simulink model "Global_Nocontrol"  (R2016a)
settings: Solver=ode8  StartTime=0.0  StopTime=1400  FixedStep=1  RelTol=1e-3
(part 1 of 2)
settings Model: Creator=Abhiram  LastModifiedBy=Abhiram
settings GRTTargetCC: GeneratePreprocessorConditionals=Use local settings

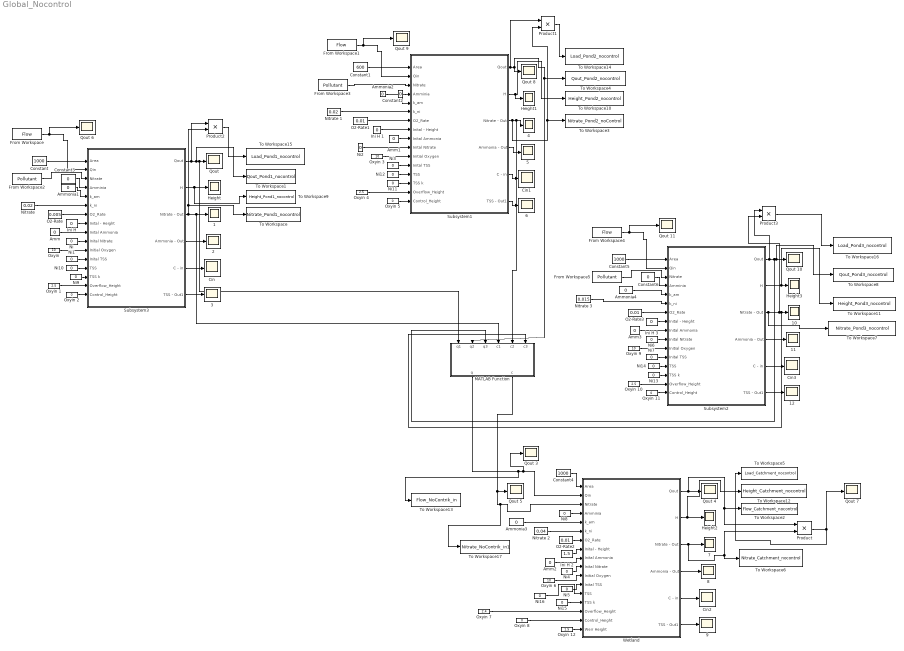
== system Global_Nocontrol ==
   Amm{,1..3} (4 alike) : Constant  Value=0
  {1..12} (12 alike) : Scope
  Ammonia{1..4} (4 alike) : Constant  Value=0
  Cin{,1..3} (4 alike) : Scope
  Constant : Constant  Value=1000
  Constant1 : Constant  Value=600
  Constant2 : Constant  Value=0
  Constant3 : Constant  Value=0
  Constant4 : Constant  Value=1000
  Constant5 : Constant  Value=1000
  Constant6 : Constant  Value=0
  From Workspace : FromWorkspace  VariableName=Flow  SampleTime=0
  From Workspace1 : FromWorkspace  VariableName=Flow  SampleTime=0
  From Workspace2 : FromWorkspace  VariableName=Pollutant  SampleTime=0
  From Workspace3 : FromWorkspace  VariableName=Pollutant  SampleTime=0
  From Workspace4 : FromWorkspace  VariableName=Flow  SampleTime=0
  From Workspace5 : FromWorkspace  VariableName=Pollutant  SampleTime=0
  Height{,1..3} (4 alike) : Scope
  "Ini H " : Constant  Value=0
  Ini H 1 : Constant  Value=0
  Ini H 2 : Constant  Value=1.5
  Ini H 3 : Constant  Value=0
  MATLAB Function : MATLAB Function  TreatAsAtomicUnit=on
  Ni{,1..16} (17 alike) : Constant  Value=0
  "Nitrate " : Constant  Value=0.02
  Nitrate 1 : Constant  Value=0.02
  Nitrate 2 : Constant  Value=0.04
  Nitrate 3 : Constant  Value=0.015
  O2-Rate : Constant  Value=0.005
  O2-Rate1 : Constant  Value=0.01
  O2-Rate2 : Constant  Value=0.01
  O2-Rate3 : Constant  Value=0.01
  Oxyin {,3,6,9} (4 alike) : Constant  Value=10
  Oxyin 1 : Constant  Value=2.5
  Oxyin 10 : Constant  Value=2.5
  Oxyin {2,5,8,11} (4 alike) : Constant  Value=0
  Oxyin 12 : Constant  Value=1.5
  Oxyin 4 : Constant  Value=2.5
  Oxyin 7 : Constant  Value=2.4
  Product{,1..3} (4 alike) : Product
  Qout {,3..11} (10 alike) : Scope
  Subsystem1 : Subsystem
  Subsystem2 : Subsystem
  Subsystem3 : Subsystem
  To Workspace : ToWorkspace  VariableName=Nitrate_Pond1_nocontrol  SampleTime=-1
      settings: Save2DSignal=2-D array (concatenate along first dimension)
  To Workspace1 : ToWorkspace  VariableName=Qout_Pond1_nocontrol  SampleTime=-1
      settings: Save2DSignal=2-D array (concatenate along first dimension)
  To Workspace10 : ToWorkspace  VariableName=Height_Pond2_nocontrol  SampleTime=-1
      settings: Save2DSignal=2-D array (concatenate along first dimension)
  To Workspace11 : ToWorkspace  VariableName=Height_Pond3_nocontrol  SampleTime=-1
      settings: Save2DSignal=2-D array (concatenate along first dimension)
  To Workspace12 : ToWorkspace  VariableName=Height_Catchment_nocontrol  SampleTime=-1
      settings: Save2DSignal=2-D array (concatenate along first dimension)
  To Workspace13 : ToWorkspace  VariableName=Flow_NoContrik_in  SampleTime=-1
      settings: Save2DSignal=2-D array (concatenate along first dimension)
  To Workspace14 : ToWorkspace  VariableName=Load_Pond2_nocontrol  SampleTime=-1
      settings: Save2DSignal=2-D array (concatenate along first dimension)
  To Workspace15 : ToWorkspace  VariableName=Load_Pond1_nocontrol  SampleTime=-1
      settings: Save2DSignal=2-D array (concatenate along first dimension)
  To Workspace16 : ToWorkspace  VariableName=Load_Pond3_nocontrol  SampleTime=-1
      settings: Save2DSignal=2-D array (concatenate along first dimension)
  To Workspace17 : ToWorkspace  VariableName=Nitrate_NoContrik_in1  SampleTime=-1
      settings: Save2DSignal=2-D array (concatenate along first dimension)
  To Workspace2 : ToWorkspace  VariableName=Flow_Catchment_nocontrol  SampleTime=-1
      settings: Save2DSignal=2-D array (concatenate along first dimension)
  To Workspace3 : ToWorkspace  VariableName=Nitrate_Pond2_noControl  SampleTime=-1
      settings: Save2DSignal=2-D array (concatenate along first dimension)
  To Workspace4 : ToWorkspace  VariableName=Qout_Pond2_nocontrol  SampleTime=-1
      settings: Save2DSignal=2-D array (concatenate along first dimension)
  To Workspace5 : ToWorkspace  VariableName=Load_Catchment_nocontrol  SampleTime=-1
      settings: Save2DSignal=2-D array (concatenate along first dimension)
  To Workspace6 : ToWorkspace  VariableName=Nitrate_Catchment_nocontrol  SampleTime=-1
      settings: Save2DSignal=2-D array (concatenate along first dimension)
  To Workspace7 : ToWorkspace  VariableName=Nitrate_Pond3_nocontrol  SampleTime=-1
      settings: Save2DSignal=2-D array (concatenate along first dimension)
  To Workspace8 : ToWorkspace  VariableName=Qout_Pond3_nocontrol  SampleTime=-1
      settings: Save2DSignal=2-D array (concatenate along first dimension)
  To Workspace9 : ToWorkspace  VariableName=Height_Pond1_nocontrol  SampleTime=-1
      settings: Save2DSignal=2-D array (concatenate along first dimension)
  Wetland : Subsystem
  wires:
  "Nitrate "/1 -> Subsystem3/6(k_ni)
  Constant/1 -> Subsystem3/1(Area)
  Ammonia1/1 -> Subsystem3/5(k_am)
  From Workspace2/1 -> Subsystem3/3(Nitrate)
  Constant3/1 -> Subsystem3/4(Amminia)
  O2-Rate/1 -> Subsystem3/7("O2_Rate ")
  Subsystem3/5("C - in ") -> Cin/1
  "Ini H "/1 -> Subsystem3/8(Inital - Height)
  " Amm"/1 -> Subsystem3/9(Inital Ammonia)
  Ni/1 -> Subsystem3/10(Inital Nitrate)
  "Oxyin "/1 -> Subsystem3/11(Initial Oxygen)
  Subsystem3/6(TSS - Out1) -> 3/1
  Ni1/1 -> Subsystem3/12(Inital TSS)
  From Workspace/1 -> Subsystem3/2(Qin), Qout 6/1
  Oxyin 1/1 -> Subsystem3/15(Overflow_Height)
  Oxyin 2/1 -> Subsystem3/16(Control_Height)
  Subsystem3/4(Ammonia - Out) -> 2/1
  Nitrate 2/1 -> Wetland/6(k_ni)
  Constant4/1 -> Wetland/1(Area)
  Ammonia3/1 -> Wetland/5(k_am)
  O2-Rate2/1 -> Wetland/7("O2_Rate ")
  Wetland/4(Ammonia - Out) -> 8/1
  Wetland/5("C - in ") -> Cin2/1
  Ini H 2/1 -> Wetland/8(Inital - Height)
  " Amm2"/1 -> Wetland/9(Inital Ammonia)
  Ni4/1 -> Wetland/10(Inital Nitrate)
  Oxyin 6/1 -> Wetland/11(Initial Oxygen)
  Wetland/6(TSS - Out1) -> 9/1
  Ni5/1 -> Wetland/12(Inital TSS)
  Oxyin 7/1 -> Wetland/15(Overflow_Height)
  Oxyin 8/1 -> Wetland/16(Control_Height)
  Wetland/3(Nitrate - Out) -> 7/1, Product/2, To Workspace6/1
  Wetland/1(Qout) -> Product/1, To Workspace2/1, Qout 4/1
  Product/1 -> Qout 7/1, To Workspace5/1
  MATLAB Function/2(c) -> To Workspace17/1, Wetland/3(Nitrate), Qout 5/1
  Ni8/1 -> Wetland/4(Amminia)
  Oxyin 12/1 -> Wetland/17(Weir Height)
  Nitrate 1/1 -> Subsystem1/6(k_ni)
  Constant1/1 -> Subsystem1/1(Area)
  Ammonia2/1 -> Subsystem1/5(k_am)
  From Workspace3/1 -> Subsystem1/3(Nitrate)
  Constant2/1 -> Subsystem1/4(Amminia)
  O2-Rate1/1 -> Subsystem1/7("O2_Rate ")
  Subsystem1/5("C - in ") -> Cin1/1
  Ini H 1/1 -> Subsystem1/8(Inital - Height)
  " Amm1"/1 -> Subsystem1/9(Inital Ammonia)
  Ni2/1 -> Subsystem1/10(Inital Nitrate)
  Oxyin 3/1 -> Subsystem1/11(Initial Oxygen)
  Subsystem1/6(TSS - Out1) -> 6/1
  Ni3/1 -> Subsystem1/12(Inital TSS)
  From Workspace1/1 -> Subsystem1/2(Qin), Qout 9/1
  Oxyin 4/1 -> Subsystem1/15(Overflow_Height)
  Oxyin 5/1 -> Subsystem1/16(Control_Height)
  Subsystem1/3(Nitrate - Out) -> To Workspace3/1, Product1/2, MATLAB Function/5(c2), 4/1
  Subsystem1/4(Ammonia - Out) -> 5/1
  Nitrate 3/1 -> Subsystem2/6(k_ni)
  Constant5/1 -> Subsystem2/1(Area)
  Ammonia4/1 -> Subsystem2/5(k_am)
  From Workspace5/1 -> Subsystem2/3(Nitrate)
  Constant6/1 -> Subsystem2/4(Amminia)
  O2-Rate3/1 -> Subsystem2/7("O2_Rate ")
  Subsystem2/5("C - in ") -> Cin3/1
  Ini H 3/1 -> Subsystem2/8(Inital - Height)
  " Amm3"/1 -> Subsystem2/9(Inital Ammonia)
  Ni6/1 -> Subsystem2/10(Inital Nitrate)
  Oxyin 9/1 -> Subsystem2/11(Initial Oxygen)
  Subsystem2/6(TSS - Out1) -> 12/1
  Ni7/1 -> Subsystem2/12(Inital TSS)
  From Workspace4/1 -> Subsystem2/2(Qin), Qout 11/1
  Oxyin 10/1 -> Subsystem2/15(Overflow_Height)
  Oxyin 11/1 -> Subsystem2/16(Control_Height)
  Subsystem2/4(Ammonia - Out) -> 11/1
  Ni9/1 -> Subsystem3/14("TSS k ")
  Ni10/1 -> Subsystem3/13(TSS)
  Ni11/1 -> Subsystem1/14("TSS k ")
  Ni12/1 -> Subsystem1/13(TSS)
  Ni13/1 -> Subsystem2/14("TSS k ")
  Ni14/1 -> Subsystem2/13(TSS)
  Ni15/1 -> Wetland/14("TSS k ")
  Ni16/1 -> Wetland/13(TSS)
  Subsystem3/2(H) -> To Workspace9/1, Height/1
  Subsystem1/2(H) -> To Workspace10/1, Height1/1
  Subsystem2/2(H) -> To Workspace11/1, Height3/1
  Wetland/2(H) -> To Workspace12/1, Height2/1
  MATLAB Function/1(q) -> To Workspace13/1, Qout 3/1, Wetland/2(Qin)
  Subsystem2/1(Qout) -> Product3/1, MATLAB Function/3(q3), To Workspace8/1, Qout 10/1
  Subsystem2/3(Nitrate - Out) -> MATLAB Function/6(c3), 10/1, Product3/2, To Workspace7/1
  Product3/1 -> To Workspace16/1
  Subsystem1/1(Qout) -> Product1/1, Qout 8/1, MATLAB Function/2(q2), To Workspace4/1
  Product1/1 -> To Workspace14/1
  Subsystem3/1(Qout) -> Product2/1, MATLAB Function/1(q1), "Qout "/1, To Workspace1/1
  Subsystem3/3(Nitrate - Out) -> Product2/2, To Workspace/1, MATLAB Function/4(c1), 1/1
  Product2/1 -> To Workspace15/1

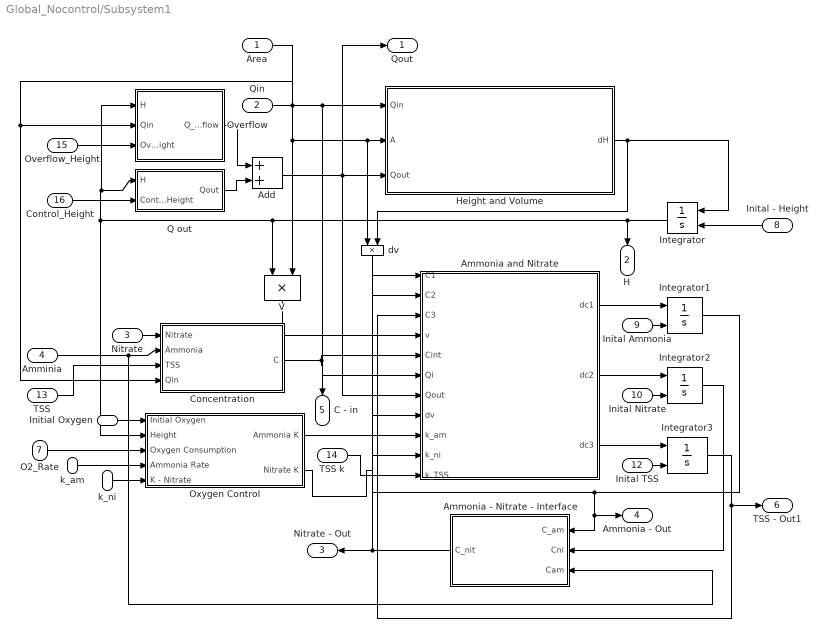
== system Global_Nocontrol/Subsystem1 ==
  Area : Inport
  Qin : Inport  Port=2
  Nitrate : Inport  Port=3
  Amminia : Inport  Port=4
  k_am : Inport  Port=5
  k_ni : Inport  Port=6
  "O2_Rate " : Inport  Port=7
  Inital - Height : Inport  Port=8
  Inital Ammonia : Inport  Port=9
  Inital Nitrate : Inport  Port=10
  Initial Oxygen : Inport  Port=11
  Inital TSS : Inport  Port=12
  TSS : Inport  Port=13
  "TSS k " : Inport  Port=14
  Overflow_Height : Inport  Port=15
  Control_Height : Inport  Port=16
  " Ammonia - Nitrate - Interface" : MATLAB Function  TreatAsAtomicUnit=on
  " Ammonia and Nitrate " : MATLAB Function  TreatAsAtomicUnit=on
  " Concentration " : MATLAB Function  TreatAsAtomicUnit=on
  Add : Sum
  Height and Volume : MATLAB Function  TreatAsAtomicUnit=on
  Integrator : Integrator  InitialConditionSource=external  InitialCondition=10  LimitOutput=on  LowerSaturationLimit=0
  Integrator1 : Integrator  InitialConditionSource=external  LimitOutput=on  LowerSaturationLimit=0
  Integrator2 : Integrator  InitialConditionSource=external  LimitOutput=on  LowerSaturationLimit=0
  Integrator3 : Integrator  InitialConditionSource=external  LimitOutput=on  LowerSaturationLimit=0
  "Overflow " : MATLAB Function  TreatAsAtomicUnit=on
  Oxygen Control : Subsystem
  Q out : MATLAB Function  TreatAsAtomicUnit=on
  V : Product
  dv : Product
  Qout : Outport
  H : Outport  Port=2
  Nitrate - Out : Outport  Port=3
  Ammonia - Out : Outport  Port=4
  "C - in " : Outport  Port=5
  TSS - Out1 : Outport  Port=6
  wires:
  Integrator2/1 -> " Ammonia - Nitrate - Interface"/2(Cni)
  " Ammonia and Nitrate "/2(dc2) -> Integrator2/1
  " Ammonia - Nitrate - Interface"/1(C_nit) -> " Ammonia and Nitrate "/2(C2), Nitrate - Out/1
  Qin/1 -> "Overflow "/2(Qin), " Concentration "/4(Qin), " Ammonia and Nitrate "/6(Qi), Height and Volume/1(Qin)
  Height and Volume/1(dH) -> Integrator/1, dv/2
  Integrator/1 -> Oxygen Control/2(Height), "Overflow "/1(H), Q out/1(H), V/1, H/1
  Add/1 -> " Ammonia and Nitrate "/7(Qout), Qout/1, Height and Volume/3(Qout)
  Amminia/1 -> " Ammonia - Nitrate - Interface"/3(Cam), " Concentration "/2(Ammonia)
  Nitrate/1 -> " Concentration "/1(Nitrate)
  V/1 -> " Ammonia and Nitrate "/4(v)
  " Ammonia and Nitrate "/1(dc1) -> Integrator1/1
  dv/1 -> " Ammonia and Nitrate "/8(dv)
  Area/1 -> V/2, dv/1, Height and Volume/2(A)
  k_am/1 -> Oxygen Control/4("Ammonia Rate ")
  Integrator1/1 -> " Ammonia - Nitrate - Interface"/1(C_am), Ammonia - Out/1, " Ammonia and Nitrate "/1(C1)
  " Concentration "/1(C) -> " Ammonia and Nitrate "/5(Cint), "C - in "/1
  Inital Ammonia/1 -> Integrator1/2
  Inital Nitrate/1 -> Integrator2/2
  Inital - Height/1 -> Integrator/2
  Oxygen Control/2(Nitrate K) -> " Ammonia and Nitrate "/10(k_ni)
  Oxygen Control/1(Ammonia K) -> " Ammonia and Nitrate "/9(k_am)
  "O2_Rate "/1 -> Oxygen Control/3(Oxygen Consumption)
  k_ni/1 -> Oxygen Control/5(K - Nitrate)
  Initial Oxygen/1 -> Oxygen Control/1(Initial Oxygen)
  Q out/1(Qout) -> Add/2
  "Overflow "/1(Q_overflow) -> Add/1
  " Ammonia and Nitrate "/3(dc3) -> Integrator3/1
  Inital TSS/1 -> Integrator3/2
  Integrator3/1 -> " Ammonia and Nitrate "/3(C3), TSS - Out1/1
  TSS/1 -> " Concentration "/3(TSS)
  "TSS k "/1 -> " Ammonia and Nitrate "/11(k_TSS)
  Overflow_Height/1 -> "Overflow "/3(Overflow_Height)
  Control_Height/1 -> Q out/2(Control_Height)

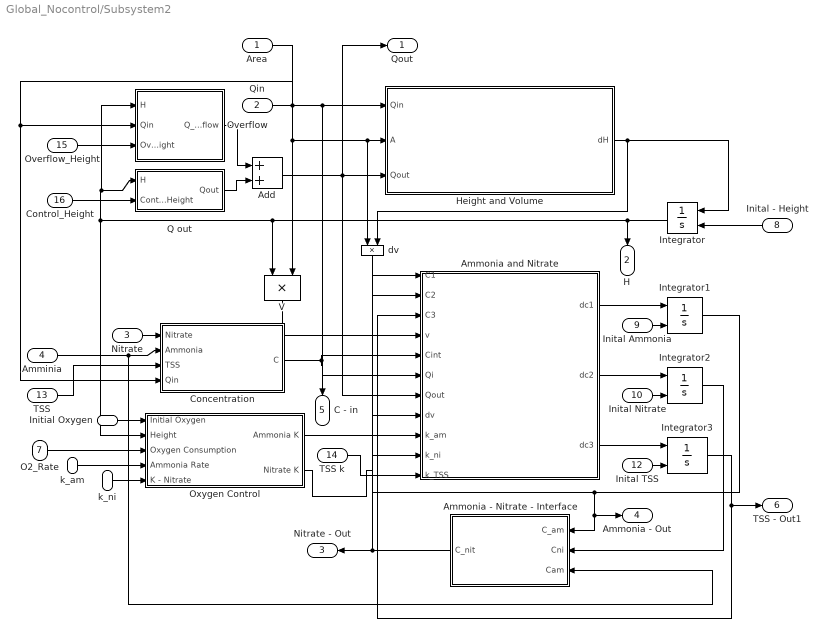
== system Global_Nocontrol/Subsystem2 ==
  Area : Inport
  Qin : Inport  Port=2
  Nitrate : Inport  Port=3
  Amminia : Inport  Port=4
  k_am : Inport  Port=5
  k_ni : Inport  Port=6
  "O2_Rate " : Inport  Port=7
  Inital - Height : Inport  Port=8
  Inital Ammonia : Inport  Port=9
  Inital Nitrate : Inport  Port=10
  Initial Oxygen : Inport  Port=11
  Inital TSS : Inport  Port=12
  TSS : Inport  Port=13
  "TSS k " : Inport  Port=14
  Overflow_Height : Inport  Port=15
  Control_Height : Inport  Port=16
  " Ammonia - Nitrate - Interface" : MATLAB Function  TreatAsAtomicUnit=on
  " Ammonia and Nitrate " : MATLAB Function  TreatAsAtomicUnit=on
  " Concentration " : MATLAB Function  TreatAsAtomicUnit=on
  Add : Sum
  Height and Volume : MATLAB Function  TreatAsAtomicUnit=on
  Integrator : Integrator  InitialConditionSource=external  InitialCondition=10  LimitOutput=on  LowerSaturationLimit=0
  Integrator1 : Integrator  InitialConditionSource=external  LimitOutput=on  LowerSaturationLimit=0
  Integrator2 : Integrator  InitialConditionSource=external  LimitOutput=on  LowerSaturationLimit=0
  Integrator3 : Integrator  InitialConditionSource=external  LimitOutput=on  LowerSaturationLimit=0
  "Overflow " : MATLAB Function  TreatAsAtomicUnit=on
  Oxygen Control : Subsystem
  Q out : MATLAB Function  TreatAsAtomicUnit=on
  V : Product
  dv : Product
  Qout : Outport
  H : Outport  Port=2
  Nitrate - Out : Outport  Port=3
  Ammonia - Out : Outport  Port=4
  "C - in " : Outport  Port=5
  TSS - Out1 : Outport  Port=6
  wires:
  Integrator2/1 -> " Ammonia - Nitrate - Interface"/2(Cni)
  " Ammonia and Nitrate "/2(dc2) -> Integrator2/1
  " Ammonia - Nitrate - Interface"/1(C_nit) -> " Ammonia and Nitrate "/2(C2), Nitrate - Out/1
  Qin/1 -> "Overflow "/2(Qin), " Concentration "/4(Qin), " Ammonia and Nitrate "/6(Qi), Height and Volume/1(Qin)
  Height and Volume/1(dH) -> Integrator/1, dv/2
  Integrator/1 -> Oxygen Control/2(Height), "Overflow "/1(H), Q out/1(H), V/1, H/1
  Add/1 -> " Ammonia and Nitrate "/7(Qout), Qout/1, Height and Volume/3(Qout)
  Amminia/1 -> " Ammonia - Nitrate - Interface"/3(Cam), " Concentration "/2(Ammonia)
  Nitrate/1 -> " Concentration "/1(Nitrate)
  V/1 -> " Ammonia and Nitrate "/4(v)
  " Ammonia and Nitrate "/1(dc1) -> Integrator1/1
  dv/1 -> " Ammonia and Nitrate "/8(dv)
  Area/1 -> V/2, dv/1, Height and Volume/2(A)
  k_am/1 -> Oxygen Control/4("Ammonia Rate ")
  Integrator1/1 -> " Ammonia - Nitrate - Interface"/1(C_am), Ammonia - Out/1, " Ammonia and Nitrate "/1(C1)
  " Concentration "/1(C) -> " Ammonia and Nitrate "/5(Cint), "C - in "/1
  Inital Ammonia/1 -> Integrator1/2
  Inital Nitrate/1 -> Integrator2/2
  Inital - Height/1 -> Integrator/2
  Oxygen Control/2(Nitrate K) -> " Ammonia and Nitrate "/10(k_ni)
  Oxygen Control/1(Ammonia K) -> " Ammonia and Nitrate "/9(k_am)
  "O2_Rate "/1 -> Oxygen Control/3(Oxygen Consumption)
  k_ni/1 -> Oxygen Control/5(K - Nitrate)
  Initial Oxygen/1 -> Oxygen Control/1(Initial Oxygen)
  Q out/1(Qout) -> Add/2
  "Overflow "/1(Q_overflow) -> Add/1
  " Ammonia and Nitrate "/3(dc3) -> Integrator3/1
  Inital TSS/1 -> Integrator3/2
  Integrator3/1 -> " Ammonia and Nitrate "/3(C3), TSS - Out1/1
  TSS/1 -> " Concentration "/3(TSS)
  "TSS k "/1 -> " Ammonia and Nitrate "/11(k_TSS)
  Overflow_Height/1 -> "Overflow "/3(Overflow_Height)
  Control_Height/1 -> Q out/2(Control_Height)

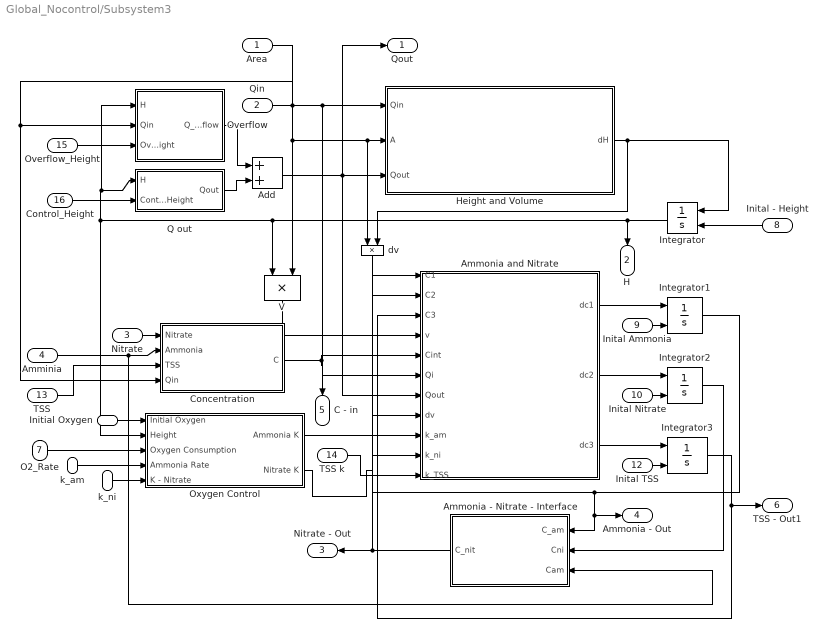
== system Global_Nocontrol/Subsystem3 ==
  Area : Inport
  Qin : Inport  Port=2
  Nitrate : Inport  Port=3
  Amminia : Inport  Port=4
  k_am : Inport  Port=5
  k_ni : Inport  Port=6
  "O2_Rate " : Inport  Port=7
  Inital - Height : Inport  Port=8
  Inital Ammonia : Inport  Port=9
  Inital Nitrate : Inport  Port=10
  Initial Oxygen : Inport  Port=11
  Inital TSS : Inport  Port=12
  TSS : Inport  Port=13
  "TSS k " : Inport  Port=14
  Overflow_Height : Inport  Port=15
  Control_Height : Inport  Port=16
  " Ammonia - Nitrate - Interface" : MATLAB Function  TreatAsAtomicUnit=on
  " Ammonia and Nitrate " : MATLAB Function  TreatAsAtomicUnit=on
  " Concentration " : MATLAB Function  TreatAsAtomicUnit=on
  Add : Sum
  Height and Volume : MATLAB Function  TreatAsAtomicUnit=on
  Integrator : Integrator  InitialConditionSource=external  InitialCondition=10  LimitOutput=on  LowerSaturationLimit=0
  Integrator1 : Integrator  InitialConditionSource=external  LimitOutput=on  LowerSaturationLimit=0
  Integrator2 : Integrator  InitialConditionSource=external  LimitOutput=on  LowerSaturationLimit=0
  Integrator3 : Integrator  InitialConditionSource=external  LimitOutput=on  LowerSaturationLimit=0
  "Overflow " : MATLAB Function  TreatAsAtomicUnit=on
  Oxygen Control : Subsystem
  Q out : MATLAB Function  TreatAsAtomicUnit=on
  V : Product
  dv : Product
  Qout : Outport
  H : Outport  Port=2
  Nitrate - Out : Outport  Port=3
  Ammonia - Out : Outport  Port=4
  "C - in " : Outport  Port=5
  TSS - Out1 : Outport  Port=6
  wires:
  Integrator2/1 -> " Ammonia - Nitrate - Interface"/2(Cni)
  " Ammonia and Nitrate "/2(dc2) -> Integrator2/1
  " Ammonia - Nitrate - Interface"/1(C_nit) -> " Ammonia and Nitrate "/2(C2), Nitrate - Out/1
  Qin/1 -> "Overflow "/2(Qin), " Concentration "/4(Qin), " Ammonia and Nitrate "/6(Qi), Height and Volume/1(Qin)
  Height and Volume/1(dH) -> Integrator/1, dv/2
  Integrator/1 -> Oxygen Control/2(Height), "Overflow "/1(H), Q out/1(H), V/1, H/1
  Add/1 -> " Ammonia and Nitrate "/7(Qout), Qout/1, Height and Volume/3(Qout)
  Amminia/1 -> " Ammonia - Nitrate - Interface"/3(Cam), " Concentration "/2(Ammonia)
  Nitrate/1 -> " Concentration "/1(Nitrate)
  V/1 -> " Ammonia and Nitrate "/4(v)
  " Ammonia and Nitrate "/1(dc1) -> Integrator1/1
  dv/1 -> " Ammonia and Nitrate "/8(dv)
  Area/1 -> V/2, dv/1, Height and Volume/2(A)
  k_am/1 -> Oxygen Control/4("Ammonia Rate ")
  Integrator1/1 -> " Ammonia - Nitrate - Interface"/1(C_am), Ammonia - Out/1, " Ammonia and Nitrate "/1(C1)
  " Concentration "/1(C) -> " Ammonia and Nitrate "/5(Cint), "C - in "/1
  Inital Ammonia/1 -> Integrator1/2
  Inital Nitrate/1 -> Integrator2/2
  Inital - Height/1 -> Integrator/2
  Oxygen Control/2(Nitrate K) -> " Ammonia and Nitrate "/10(k_ni)
  Oxygen Control/1(Ammonia K) -> " Ammonia and Nitrate "/9(k_am)
  "O2_Rate "/1 -> Oxygen Control/3(Oxygen Consumption)
  k_ni/1 -> Oxygen Control/5(K - Nitrate)
  Initial Oxygen/1 -> Oxygen Control/1(Initial Oxygen)
  Q out/1(Qout) -> Add/2
  "Overflow "/1(Q_overflow) -> Add/1
  " Ammonia and Nitrate "/3(dc3) -> Integrator3/1
  Inital TSS/1 -> Integrator3/2
  Integrator3/1 -> " Ammonia and Nitrate "/3(C3), TSS - Out1/1
  TSS/1 -> " Concentration "/3(TSS)
  "TSS k "/1 -> " Ammonia and Nitrate "/11(k_TSS)
  Overflow_Height/1 -> "Overflow "/3(Overflow_Height)
  Control_Height/1 -> Q out/2(Control_Height)

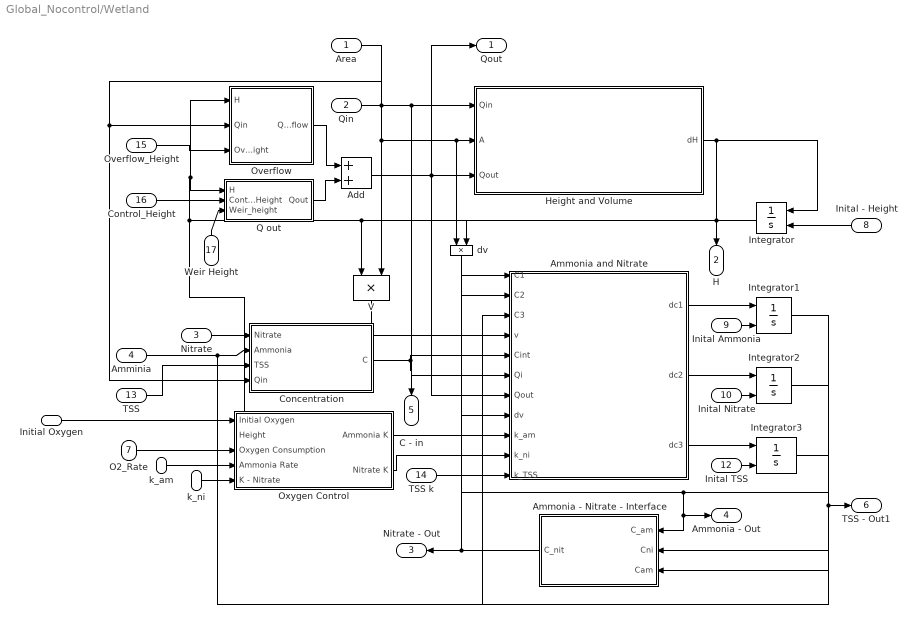
== system Global_Nocontrol/Wetland ==
  Area : Inport
  Qin : Inport  Port=2
  Nitrate : Inport  Port=3
  Amminia : Inport  Port=4
  k_am : Inport  Port=5
  k_ni : Inport  Port=6
  "O2_Rate " : Inport  Port=7
  Inital - Height : Inport  Port=8
  Inital Ammonia : Inport  Port=9
  Inital Nitrate : Inport  Port=10
  Initial Oxygen : Inport  Port=11
  Inital TSS : Inport  Port=12
  TSS : Inport  Port=13
  "TSS k " : Inport  Port=14
  Overflow_Height : Inport  Port=15
  Control_Height : Inport  Port=16
  Weir Height : Inport  Port=17
  " Ammonia - Nitrate - Interface" : MATLAB Function  TreatAsAtomicUnit=on
  " Ammonia and Nitrate " : MATLAB Function  TreatAsAtomicUnit=on
  " Concentration " : MATLAB Function  TreatAsAtomicUnit=on
  Add : Sum
  Height and Volume : MATLAB Function  TreatAsAtomicUnit=on
  Integrator : Integrator  InitialConditionSource=external  InitialCondition=10  LimitOutput=on  LowerSaturationLimit=0
  Integrator1 : Integrator  InitialConditionSource=external  LimitOutput=on  LowerSaturationLimit=0
  Integrator2 : Integrator  InitialConditionSource=external  LimitOutput=on  LowerSaturationLimit=0
  Integrator3 : Integrator  InitialConditionSource=external  LimitOutput=on  LowerSaturationLimit=0
  "Overflow " : MATLAB Function  TreatAsAtomicUnit=on
  Oxygen Control : Subsystem
  Q out : MATLAB Function  TreatAsAtomicUnit=on
  V : Product
  dv : Product
  Qout : Outport
  H : Outport  Port=2
  Nitrate - Out : Outport  Port=3
  Ammonia - Out : Outport  Port=4
  "C - in " : Outport  Port=5
  TSS - Out1 : Outport  Port=6
  wires:
  Integrator2/1 -> " Ammonia - Nitrate - Interface"/2(Cni)
  " Ammonia and Nitrate "/2(dc2) -> Integrator2/1
  " Ammonia - Nitrate - Interface"/1(C_nit) -> " Ammonia and Nitrate "/2(C2), Nitrate - Out/1
  Qin/1 -> "Overflow "/2(Qin), " Concentration "/4(Qin), " Ammonia and Nitrate "/6(Qi), Height and Volume/1(Qin)
  Height and Volume/1(dH) -> Integrator/1, dv/2
  Integrator/1 -> Oxygen Control/2(Height), Q out/1(H), "Overflow "/1(H), V/1, H/1
  Add/1 -> " Ammonia and Nitrate "/7(Qout), Qout/1, Height and Volume/3(Qout)
  Amminia/1 -> " Ammonia - Nitrate - Interface"/3(Cam), " Concentration "/2(Ammonia)
  Nitrate/1 -> " Concentration "/1(Nitrate)
  V/1 -> " Ammonia and Nitrate "/4(v)
  " Ammonia and Nitrate "/1(dc1) -> Integrator1/1
  dv/1 -> " Ammonia and Nitrate "/8(dv)
  Area/1 -> V/2, dv/1, Height and Volume/2(A)
  k_am/1 -> Oxygen Control/4("Ammonia Rate ")
  Integrator1/1 -> " Ammonia - Nitrate - Interface"/1(C_am), Ammonia - Out/1, " Ammonia and Nitrate "/1(C1)
  " Concentration "/1(C) -> "C - in "/1, " Ammonia and Nitrate "/5(Cint)
  Inital Ammonia/1 -> Integrator1/2
  Inital Nitrate/1 -> Integrator2/2
  Inital - Height/1 -> Integrator/2
  Oxygen Control/2(Nitrate K) -> " Ammonia and Nitrate "/10(k_ni)
  "O2_Rate "/1 -> Oxygen Control/3(Oxygen Consumption)
  k_ni/1 -> Oxygen Control/5(K - Nitrate)
  Initial Oxygen/1 -> Oxygen Control/1(Initial Oxygen)
  Q out/1(Qout) -> Add/2
  "Overflow "/1(Q_overflow) -> Add/1
  " Ammonia and Nitrate "/3(dc3) -> Integrator3/1
  Inital TSS/1 -> Integrator3/2
  Integrator3/1 -> " Ammonia and Nitrate "/3(C3), TSS - Out1/1
  TSS/1 -> " Concentration "/3(TSS)
  "TSS k "/1 -> " Ammonia and Nitrate "/11(k_TSS)
  Overflow_Height/1 -> "Overflow "/3(Overflow_Height)
  Control_Height/1 -> Q out/2(Control_Height)
  Oxygen Control/1(Ammonia K) -> " Ammonia and Nitrate "/9(k_am)
  Weir Height/1 -> Q out/3(Weir_height)

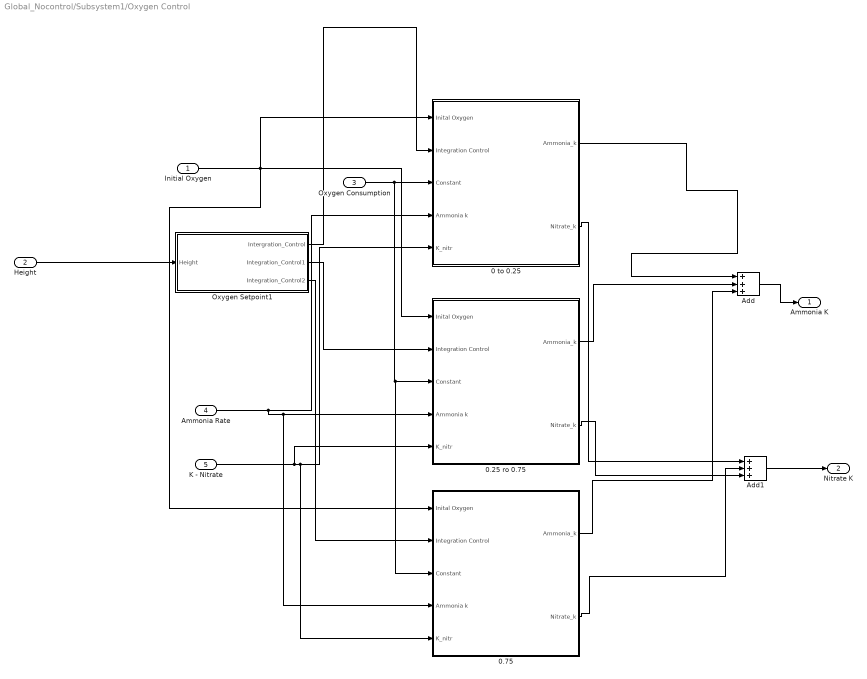
== system Global_Nocontrol/Subsystem1/Oxygen Control ==
  Initial Oxygen : Inport
  Height : Inport  Port=2
  Oxygen Consumption : Inport  Port=3
  "Ammonia Rate " : Inport  Port=4
  K - Nitrate : Inport  Port=5
  " Oxygen Setpoint1" : MATLAB Function  TreatAsAtomicUnit=on
  0 to 0.25 : Subsystem
  0.25 ro 0.75 : Subsystem
  "0.75 " : Subsystem
  Add : Sum  Inputs=3
  Add1 : Sum  Inputs=3
  Ammonia K : Outport
  Nitrate K : Outport  Port=2
  wires:
  Height/1 -> " Oxygen Setpoint1"/1(Height)
  " Oxygen Setpoint1"/2(Integration_Control1) -> 0.25 ro 0.75/2(Integration Control)
  " Oxygen Setpoint1"/1(Intergration_Control) -> 0 to 0.25/2(Integration Control)
  0 to 0.25/1(Ammonia_k) -> Add/1
  0 to 0.25/2("Nitrate_k ") -> Add1/1
  0.25 ro 0.75/1(Ammonia_k) -> Add/2
  0.25 ro 0.75/2("Nitrate_k ") -> Add1/3
  " Oxygen Setpoint1"/3(Integration_Control2) -> "0.75 "/2(Integration Control)
  Initial Oxygen/1 -> "0.75 "/1(Inital Oxygen), 0.25 ro 0.75/1(Inital Oxygen), 0 to 0.25/1(Inital Oxygen)
  Oxygen Consumption/1 -> "0.75 "/3(Constant), 0.25 ro 0.75/3(Constant), 0 to 0.25/3(Constant)
  "Ammonia Rate "/1 -> "0.75 "/4(Ammonia k), 0.25 ro 0.75/4(Ammonia k), 0 to 0.25/4(Ammonia k)
  K - Nitrate/1 -> 0.25 ro 0.75/5(K_nitr), "0.75 "/5(K_nitr), 0 to 0.25/5(K_nitr)
  "0.75 "/2("Nitrate_k ") -> Add1/2
  "0.75 "/1(Ammonia_k) -> Add/3
  Add1/1 -> Nitrate K/1
  Add/1 -> Ammonia K/1

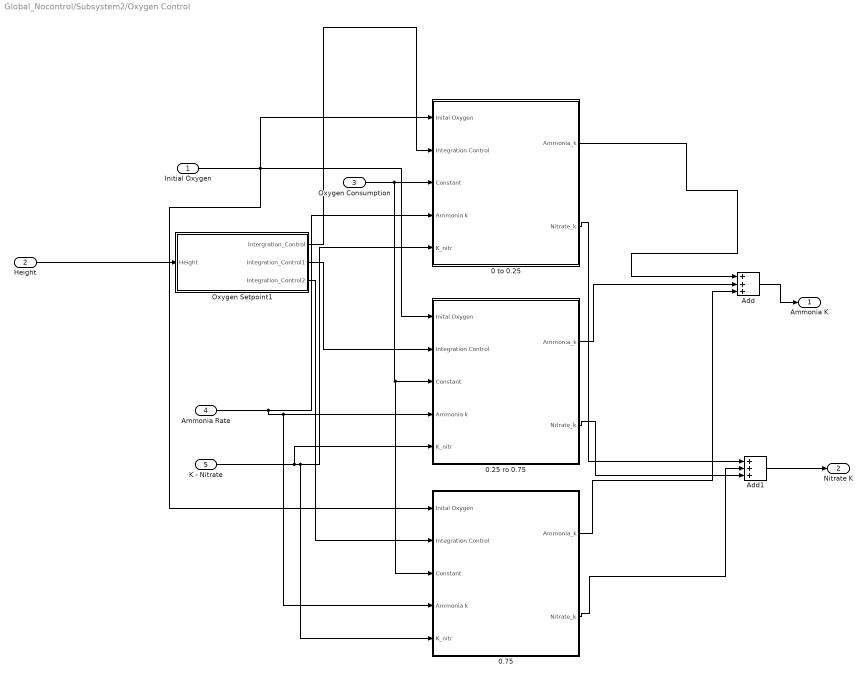
== system Global_Nocontrol/Subsystem2/Oxygen Control ==
  Initial Oxygen : Inport
  Height : Inport  Port=2
  Oxygen Consumption : Inport  Port=3
  "Ammonia Rate " : Inport  Port=4
  K - Nitrate : Inport  Port=5
  " Oxygen Setpoint1" : MATLAB Function  TreatAsAtomicUnit=on
  0 to 0.25 : Subsystem
  0.25 ro 0.75 : Subsystem
  "0.75 " : Subsystem
  Add : Sum  Inputs=3
  Add1 : Sum  Inputs=3
  Ammonia K : Outport
  Nitrate K : Outport  Port=2
  wires:
  Height/1 -> " Oxygen Setpoint1"/1(Height)
  " Oxygen Setpoint1"/2(Integration_Control1) -> 0.25 ro 0.75/2(Integration Control)
  " Oxygen Setpoint1"/1(Intergration_Control) -> 0 to 0.25/2(Integration Control)
  0 to 0.25/1(Ammonia_k) -> Add/1
  0 to 0.25/2("Nitrate_k ") -> Add1/1
  0.25 ro 0.75/1(Ammonia_k) -> Add/2
  0.25 ro 0.75/2("Nitrate_k ") -> Add1/3
  " Oxygen Setpoint1"/3(Integration_Control2) -> "0.75 "/2(Integration Control)
  Initial Oxygen/1 -> "0.75 "/1(Inital Oxygen), 0.25 ro 0.75/1(Inital Oxygen), 0 to 0.25/1(Inital Oxygen)
  Oxygen Consumption/1 -> "0.75 "/3(Constant), 0.25 ro 0.75/3(Constant), 0 to 0.25/3(Constant)
  "Ammonia Rate "/1 -> "0.75 "/4(Ammonia k), 0.25 ro 0.75/4(Ammonia k), 0 to 0.25/4(Ammonia k)
  K - Nitrate/1 -> 0.25 ro 0.75/5(K_nitr), "0.75 "/5(K_nitr), 0 to 0.25/5(K_nitr)
  "0.75 "/2("Nitrate_k ") -> Add1/2
  "0.75 "/1(Ammonia_k) -> Add/3
  Add1/1 -> Nitrate K/1
  Add/1 -> Ammonia K/1

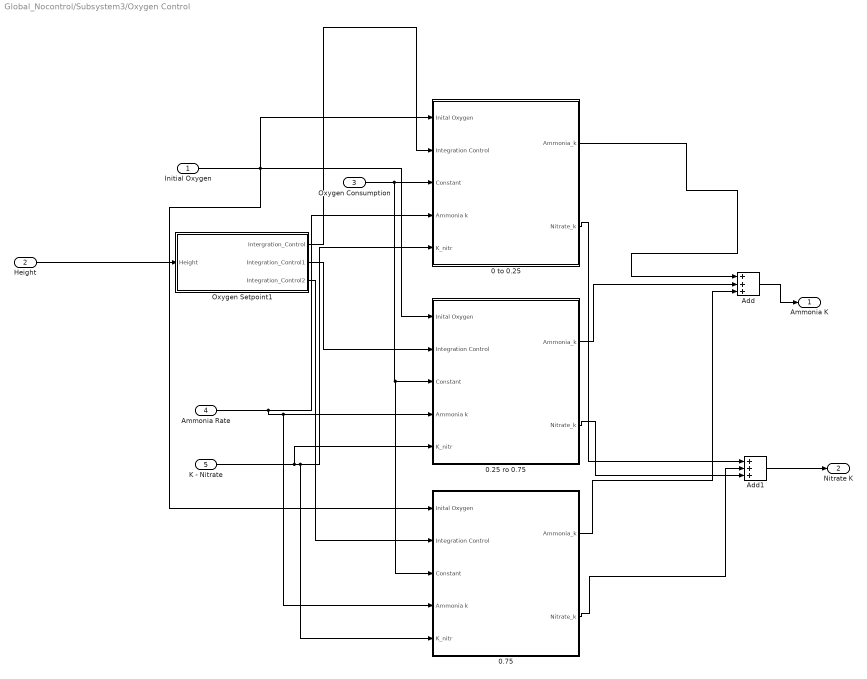
== system Global_Nocontrol/Subsystem3/Oxygen Control ==
  Initial Oxygen : Inport
  Height : Inport  Port=2
  Oxygen Consumption : Inport  Port=3
  "Ammonia Rate " : Inport  Port=4
  K - Nitrate : Inport  Port=5
  " Oxygen Setpoint1" : MATLAB Function  TreatAsAtomicUnit=on
  0 to 0.25 : Subsystem
  0.25 ro 0.75 : Subsystem
  "0.75 " : Subsystem
  Add : Sum  Inputs=3
  Add1 : Sum  Inputs=3
  Ammonia K : Outport
  Nitrate K : Outport  Port=2
  wires:
  Height/1 -> " Oxygen Setpoint1"/1(Height)
  " Oxygen Setpoint1"/2(Integration_Control1) -> 0.25 ro 0.75/2(Integration Control)
  " Oxygen Setpoint1"/1(Intergration_Control) -> 0 to 0.25/2(Integration Control)
  0 to 0.25/1(Ammonia_k) -> Add/1
  0 to 0.25/2("Nitrate_k ") -> Add1/1
  0.25 ro 0.75/1(Ammonia_k) -> Add/2
  0.25 ro 0.75/2("Nitrate_k ") -> Add1/3
  " Oxygen Setpoint1"/3(Integration_Control2) -> "0.75 "/2(Integration Control)
  Initial Oxygen/1 -> "0.75 "/1(Inital Oxygen), 0.25 ro 0.75/1(Inital Oxygen), 0 to 0.25/1(Inital Oxygen)
  Oxygen Consumption/1 -> "0.75 "/3(Constant), 0.25 ro 0.75/3(Constant), 0 to 0.25/3(Constant)
  "Ammonia Rate "/1 -> "0.75 "/4(Ammonia k), 0.25 ro 0.75/4(Ammonia k), 0 to 0.25/4(Ammonia k)
  K - Nitrate/1 -> 0.25 ro 0.75/5(K_nitr), "0.75 "/5(K_nitr), 0 to 0.25/5(K_nitr)
  "0.75 "/2("Nitrate_k ") -> Add1/2
  "0.75 "/1(Ammonia_k) -> Add/3
  Add1/1 -> Nitrate K/1
  Add/1 -> Ammonia K/1

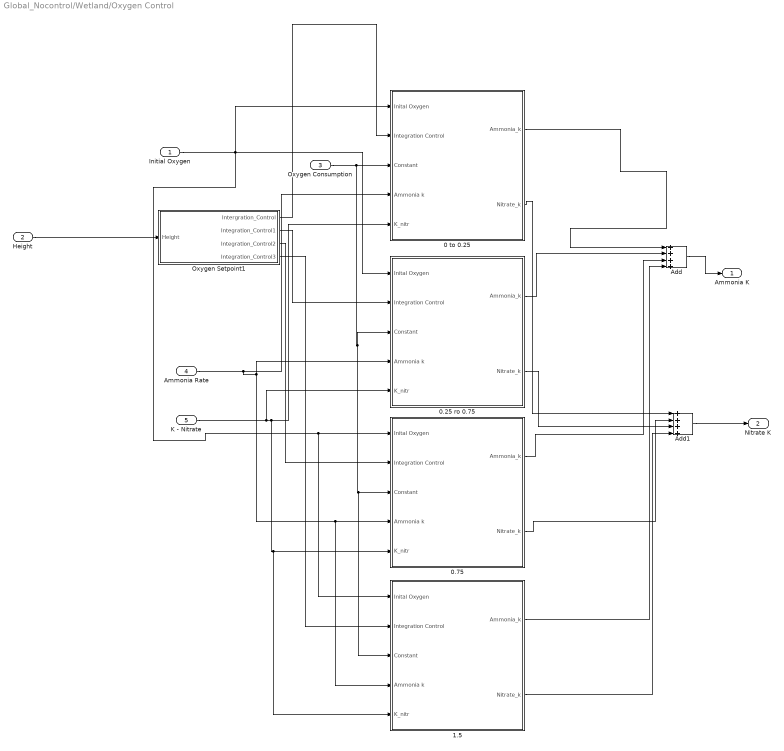
== system Global_Nocontrol/Wetland/Oxygen Control ==
  Initial Oxygen : Inport
  Height : Inport  Port=2
  Oxygen Consumption : Inport  Port=3
  "Ammonia Rate " : Inport  Port=4
  K - Nitrate : Inport  Port=5
  " 1.5" : Subsystem
  " Oxygen Setpoint1" : MATLAB Function  TreatAsAtomicUnit=on
  0 to 0.25 : Subsystem
  0.25 ro 0.75 : Subsystem
  "0.75 " : Subsystem
  Add : Sum  Inputs=4
  Add1 : Sum  Inputs=4
  Ammonia K : Outport
  Nitrate K : Outport  Port=2
  wires:
  Height/1 -> " Oxygen Setpoint1"/1(Height)
  " Oxygen Setpoint1"/2(Integration_Control1) -> 0.25 ro 0.75/2(Integration Control)
  " Oxygen Setpoint1"/1(Intergration_Control) -> 0 to 0.25/2(Integration Control)
  0 to 0.25/1(Ammonia_k) -> Add/1
  0 to 0.25/2("Nitrate_k ") -> Add1/1
  0.25 ro 0.75/1(Ammonia_k) -> Add/2
  0.25 ro 0.75/2("Nitrate_k ") -> Add1/3
  " Oxygen Setpoint1"/3(Integration_Control2) -> "0.75 "/2(Integration Control)
  Initial Oxygen/1 -> " 1.5"/1(Inital Oxygen), "0.75 "/1(Inital Oxygen), 0.25 ro 0.75/1(Inital Oxygen), 0 to 0.25/1(Inital Oxygen)
  Oxygen Consumption/1 -> " 1.5"/3(Constant), "0.75 "/3(Constant), 0.25 ro 0.75/3(Constant), 0 to 0.25/3(Constant)
  "Ammonia Rate "/1 -> " 1.5"/4(Ammonia k), "0.75 "/4(Ammonia k), 0.25 ro 0.75/4(Ammonia k), 0 to 0.25/4(Ammonia k)
  K - Nitrate/1 -> 0.25 ro 0.75/5(K_nitr), " 1.5"/5(K_nitr), "0.75 "/5(K_nitr), 0 to 0.25/5(K_nitr)
  "0.75 "/2("Nitrate_k ") -> Add1/2
  "0.75 "/1(Ammonia_k) -> Add/3
  Add1/1 -> Nitrate K/1
  Add/1 -> Ammonia K/1
  " 1.5"/1(Ammonia_k) -> Add/4
  " 1.5"/2("Nitrate_k ") -> Add1/4
  " Oxygen Setpoint1"/4(Integration_Control3) -> " 1.5"/2(Integration Control)

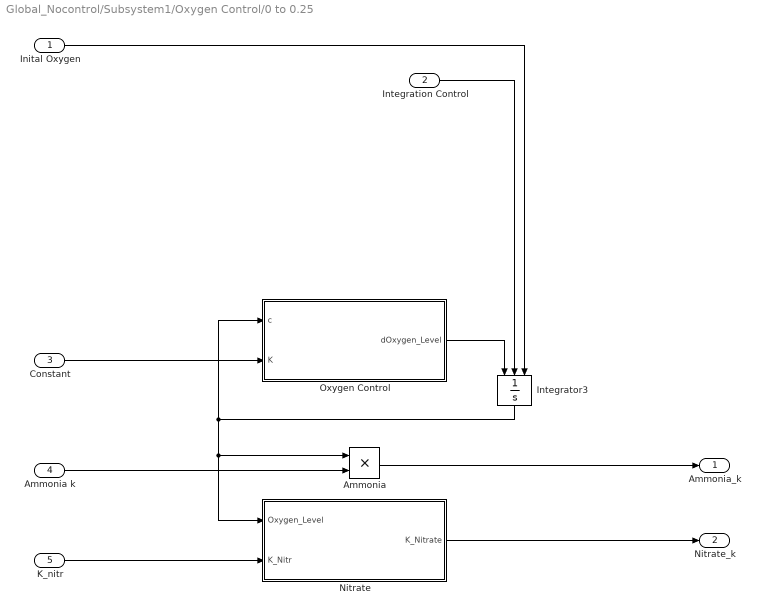
== system Global_Nocontrol/Subsystem1/Oxygen Control/0 to 0.25 ==
  Inital Oxygen : Inport
  Integration Control : Inport  Port=2
  Constant : Inport  Port=3
  Ammonia k : Inport  Port=4
  K_nitr : Inport  Port=5
  " Nitrate" : MATLAB Function  TreatAsAtomicUnit=on
  " Oxygen Control" : MATLAB Function  TreatAsAtomicUnit=on
  Ammonia : Product
  Integrator3 : Integrator  ExternalReset=level hold  InitialConditionSource=external  InitialCondition=10
  Ammonia_k : Outport
  "Nitrate_k " : Outport  Port=2
  wires:
  Inital Oxygen/1 -> Integrator3/3
  " Nitrate"/1(K_Nitrate) -> "Nitrate_k "/1
  Ammonia/1 -> Ammonia_k/1
  Ammonia k/1 -> Ammonia/2
  Constant/1 -> " Oxygen Control"/2(K)
  " Oxygen Control"/1(dOxygen_Level) -> Integrator3/1
  Integrator3/1 -> " Oxygen Control"/1(c), " Nitrate"/1(Oxygen_Level), Ammonia/1
  K_nitr/1 -> " Nitrate"/2(K_Nitr)
  Integration Control/1 -> Integrator3/2

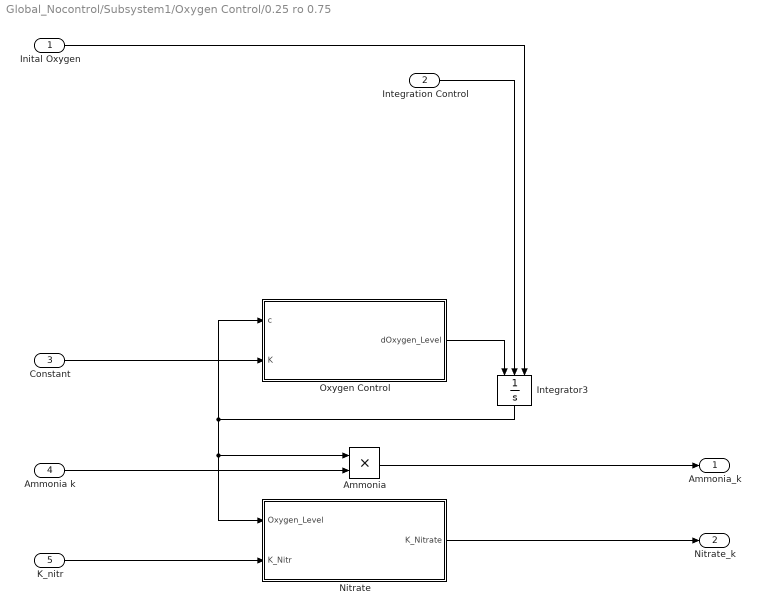
== system Global_Nocontrol/Subsystem1/Oxygen Control/0.25 ro 0.75 ==
  Inital Oxygen : Inport
  Integration Control : Inport  Port=2
  Constant : Inport  Port=3
  Ammonia k : Inport  Port=4
  K_nitr : Inport  Port=5
  " Nitrate" : MATLAB Function  TreatAsAtomicUnit=on
  " Oxygen Control" : MATLAB Function  TreatAsAtomicUnit=on
  Ammonia : Product
  Integrator3 : Integrator  ExternalReset=level hold  InitialConditionSource=external  InitialCondition=10
  Ammonia_k : Outport
  "Nitrate_k " : Outport  Port=2
  wires:
  Inital Oxygen/1 -> Integrator3/3
  " Nitrate"/1(K_Nitrate) -> "Nitrate_k "/1
  Ammonia/1 -> Ammonia_k/1
  Ammonia k/1 -> Ammonia/2
  Constant/1 -> " Oxygen Control"/2(K)
  " Oxygen Control"/1(dOxygen_Level) -> Integrator3/1
  Integrator3/1 -> " Oxygen Control"/1(c), " Nitrate"/1(Oxygen_Level), Ammonia/1
  K_nitr/1 -> " Nitrate"/2(K_Nitr)
  Integration Control/1 -> Integrator3/2

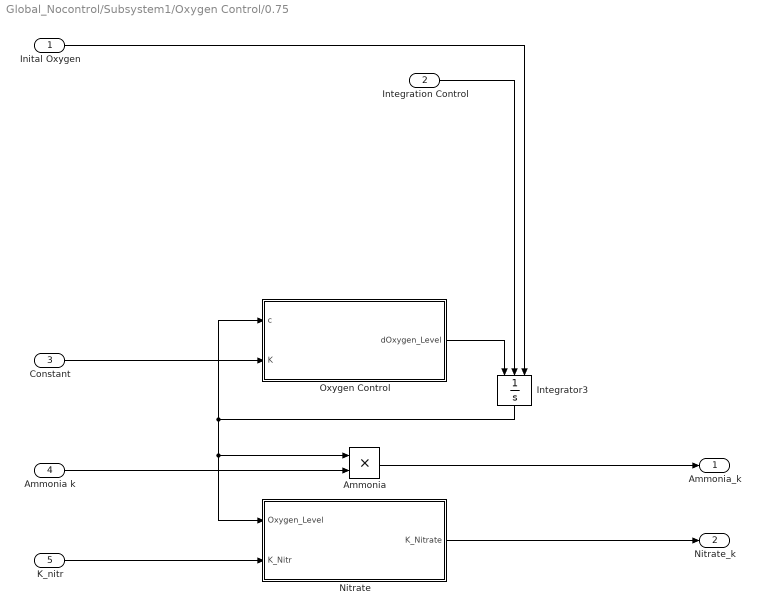
== system Global_Nocontrol/Subsystem1/Oxygen Control/0.75  ==
  Inital Oxygen : Inport
  Integration Control : Inport  Port=2
  Constant : Inport  Port=3
  Ammonia k : Inport  Port=4
  K_nitr : Inport  Port=5
  " Nitrate" : MATLAB Function  TreatAsAtomicUnit=on
  " Oxygen Control" : MATLAB Function  TreatAsAtomicUnit=on
  Ammonia : Product
  Integrator3 : Integrator  ExternalReset=level hold  InitialConditionSource=external  InitialCondition=10
  Ammonia_k : Outport
  "Nitrate_k " : Outport  Port=2
  wires:
  Inital Oxygen/1 -> Integrator3/3
  " Nitrate"/1(K_Nitrate) -> "Nitrate_k "/1
  Ammonia/1 -> Ammonia_k/1
  Ammonia k/1 -> Ammonia/2
  Constant/1 -> " Oxygen Control"/2(K)
  " Oxygen Control"/1(dOxygen_Level) -> Integrator3/1
  Integrator3/1 -> " Oxygen Control"/1(c), " Nitrate"/1(Oxygen_Level), Ammonia/1
  K_nitr/1 -> " Nitrate"/2(K_Nitr)
  Integration Control/1 -> Integrator3/2

== system Global_Nocontrol/Subsystem2/Oxygen Control/0 to 0.25 ==
  Inital Oxygen : Inport
  Integration Control : Inport  Port=2
  Constant : Inport  Port=3
  Ammonia k : Inport  Port=4
  K_nitr : Inport  Port=5
  " Nitrate" : MATLAB Function  TreatAsAtomicUnit=on
  " Oxygen Control" : MATLAB Function  TreatAsAtomicUnit=on
  Ammonia : Product
  Integrator3 : Integrator  ExternalReset=level hold  InitialConditionSource=external  InitialCondition=10
  Ammonia_k : Outport
  "Nitrate_k " : Outport  Port=2
  wires:
  Inital Oxygen/1 -> Integrator3/3
  " Nitrate"/1(K_Nitrate) -> "Nitrate_k "/1
  Ammonia/1 -> Ammonia_k/1
  Ammonia k/1 -> Ammonia/2
  Constant/1 -> " Oxygen Control"/2(K)
  " Oxygen Control"/1(dOxygen_Level) -> Integrator3/1
  Integrator3/1 -> " Oxygen Control"/1(c), " Nitrate"/1(Oxygen_Level), Ammonia/1
  K_nitr/1 -> " Nitrate"/2(K_Nitr)
  Integration Control/1 -> Integrator3/2

== system Global_Nocontrol/Subsystem2/Oxygen Control/0.25 ro 0.75 ==
  Inital Oxygen : Inport
  Integration Control : Inport  Port=2
  Constant : Inport  Port=3
  Ammonia k : Inport  Port=4
  K_nitr : Inport  Port=5
  " Nitrate" : MATLAB Function  TreatAsAtomicUnit=on
  " Oxygen Control" : MATLAB Function  TreatAsAtomicUnit=on
  Ammonia : Product
  Integrator3 : Integrator  ExternalReset=level hold  InitialConditionSource=external  InitialCondition=10
  Ammonia_k : Outport
  "Nitrate_k " : Outport  Port=2
  wires:
  Inital Oxygen/1 -> Integrator3/3
  " Nitrate"/1(K_Nitrate) -> "Nitrate_k "/1
  Ammonia/1 -> Ammonia_k/1
  Ammonia k/1 -> Ammonia/2
  Constant/1 -> " Oxygen Control"/2(K)
  " Oxygen Control"/1(dOxygen_Level) -> Integrator3/1
  Integrator3/1 -> " Oxygen Control"/1(c), " Nitrate"/1(Oxygen_Level), Ammonia/1
  K_nitr/1 -> " Nitrate"/2(K_Nitr)
  Integration Control/1 -> Integrator3/2

== system Global_Nocontrol/Subsystem2/Oxygen Control/0.75  ==
  Inital Oxygen : Inport
  Integration Control : Inport  Port=2
  Constant : Inport  Port=3
  Ammonia k : Inport  Port=4
  K_nitr : Inport  Port=5
  " Nitrate" : MATLAB Function  TreatAsAtomicUnit=on
  " Oxygen Control" : MATLAB Function  TreatAsAtomicUnit=on
  Ammonia : Product
  Integrator3 : Integrator  ExternalReset=level hold  InitialConditionSource=external  InitialCondition=10
  Ammonia_k : Outport
  "Nitrate_k " : Outport  Port=2
  wires:
  Inital Oxygen/1 -> Integrator3/3
  " Nitrate"/1(K_Nitrate) -> "Nitrate_k "/1
  Ammonia/1 -> Ammonia_k/1
  Ammonia k/1 -> Ammonia/2
  Constant/1 -> " Oxygen Control"/2(K)
  " Oxygen Control"/1(dOxygen_Level) -> Integrator3/1
  Integrator3/1 -> " Oxygen Control"/1(c), " Nitrate"/1(Oxygen_Level), Ammonia/1
  K_nitr/1 -> " Nitrate"/2(K_Nitr)
  Integration Control/1 -> Integrator3/2

== system Global_Nocontrol/Subsystem3/Oxygen Control/0 to 0.25 ==
  Inital Oxygen : Inport
  Integration Control : Inport  Port=2
  Constant : Inport  Port=3
  Ammonia k : Inport  Port=4
  K_nitr : Inport  Port=5
  " Nitrate" : MATLAB Function  TreatAsAtomicUnit=on
  " Oxygen Control" : MATLAB Function  TreatAsAtomicUnit=on
  Ammonia : Product
  Integrator3 : Integrator  ExternalReset=level hold  InitialConditionSource=external  InitialCondition=10
  Ammonia_k : Outport
  "Nitrate_k " : Outport  Port=2
  wires:
  Inital Oxygen/1 -> Integrator3/3
  " Nitrate"/1(K_Nitrate) -> "Nitrate_k "/1
  Ammonia/1 -> Ammonia_k/1
  Ammonia k/1 -> Ammonia/2
  Constant/1 -> " Oxygen Control"/2(K)
  " Oxygen Control"/1(dOxygen_Level) -> Integrator3/1
  Integrator3/1 -> " Oxygen Control"/1(c), " Nitrate"/1(Oxygen_Level), Ammonia/1
  K_nitr/1 -> " Nitrate"/2(K_Nitr)
  Integration Control/1 -> Integrator3/2

== system Global_Nocontrol/Subsystem3/Oxygen Control/0.25 ro 0.75 ==
  Inital Oxygen : Inport
  Integration Control : Inport  Port=2
  Constant : Inport  Port=3
  Ammonia k : Inport  Port=4
  K_nitr : Inport  Port=5
  " Nitrate" : MATLAB Function  TreatAsAtomicUnit=on
  " Oxygen Control" : MATLAB Function  TreatAsAtomicUnit=on
  Ammonia : Product
  Integrator3 : Integrator  ExternalReset=level hold  InitialConditionSource=external  InitialCondition=10
  Ammonia_k : Outport
  "Nitrate_k " : Outport  Port=2
  wires:
  Inital Oxygen/1 -> Integrator3/3
  " Nitrate"/1(K_Nitrate) -> "Nitrate_k "/1
  Ammonia/1 -> Ammonia_k/1
  Ammonia k/1 -> Ammonia/2
  Constant/1 -> " Oxygen Control"/2(K)
  " Oxygen Control"/1(dOxygen_Level) -> Integrator3/1
  Integrator3/1 -> " Oxygen Control"/1(c), " Nitrate"/1(Oxygen_Level), Ammonia/1
  K_nitr/1 -> " Nitrate"/2(K_Nitr)
  Integration Control/1 -> Integrator3/2

== system Global_Nocontrol/Subsystem3/Oxygen Control/0.75  ==
  Inital Oxygen : Inport
  Integration Control : Inport  Port=2
  Constant : Inport  Port=3
  Ammonia k : Inport  Port=4
  K_nitr : Inport  Port=5
  " Nitrate" : MATLAB Function  TreatAsAtomicUnit=on
  " Oxygen Control" : MATLAB Function  TreatAsAtomicUnit=on
  Ammonia : Product
  Integrator3 : Integrator  ExternalReset=level hold  InitialConditionSource=external  InitialCondition=10
  Ammonia_k : Outport
  "Nitrate_k " : Outport  Port=2
  wires:
  Inital Oxygen/1 -> Integrator3/3
  " Nitrate"/1(K_Nitrate) -> "Nitrate_k "/1
  Ammonia/1 -> Ammonia_k/1
  Ammonia k/1 -> Ammonia/2
  Constant/1 -> " Oxygen Control"/2(K)
  " Oxygen Control"/1(dOxygen_Level) -> Integrator3/1
  Integrator3/1 -> " Oxygen Control"/1(c), " Nitrate"/1(Oxygen_Level), Ammonia/1
  K_nitr/1 -> " Nitrate"/2(K_Nitr)
  Integration Control/1 -> Integrator3/2

== system Global_Nocontrol/Wetland/Oxygen Control/ 1.5 ==
  Inital Oxygen : Inport
  Integration Control : Inport  Port=2
  Constant : Inport  Port=3
  Ammonia k : Inport  Port=4
  K_nitr : Inport  Port=5
  " Nitrate" : MATLAB Function  TreatAsAtomicUnit=on
  " Oxygen Control" : MATLAB Function  TreatAsAtomicUnit=on
  Ammonia : Product
  Integrator3 : Integrator  ExternalReset=level hold  InitialConditionSource=external  InitialCondition=10
  Ammonia_k : Outport
  "Nitrate_k " : Outport  Port=2
  wires:
  Inital Oxygen/1 -> Integrator3/3
  " Nitrate"/1(K_Nitrate) -> "Nitrate_k "/1
  Ammonia/1 -> Ammonia_k/1
  Ammonia k/1 -> Ammonia/2
  Constant/1 -> " Oxygen Control"/2(K)
  " Oxygen Control"/1(dOxygen_Level) -> Integrator3/1
  Integrator3/1 -> " Oxygen Control"/1(c), " Nitrate"/1(Oxygen_Level), Ammonia/1
  K_nitr/1 -> " Nitrate"/2(K_Nitr)
  Integration Control/1 -> Integrator3/2

== system Global_Nocontrol/Wetland/Oxygen Control/0 to 0.25 ==
  Inital Oxygen : Inport
  Integration Control : Inport  Port=2
  Constant : Inport  Port=3
  Ammonia k : Inport  Port=4
  K_nitr : Inport  Port=5
  " Nitrate" : MATLAB Function  TreatAsAtomicUnit=on
  " Oxygen Control" : MATLAB Function  TreatAsAtomicUnit=on
  Ammonia : Product
  Integrator3 : Integrator  ExternalReset=level hold  InitialConditionSource=external  InitialCondition=10
  Ammonia_k : Outport
  "Nitrate_k " : Outport  Port=2
  wires:
  Inital Oxygen/1 -> Integrator3/3
  " Nitrate"/1(K_Nitrate) -> "Nitrate_k "/1
  Ammonia/1 -> Ammonia_k/1
  Ammonia k/1 -> Ammonia/2
  Constant/1 -> " Oxygen Control"/2(K)
  " Oxygen Control"/1(dOxygen_Level) -> Integrator3/1
  Integrator3/1 -> " Oxygen Control"/1(c), " Nitrate"/1(Oxygen_Level), Ammonia/1
  K_nitr/1 -> " Nitrate"/2(K_Nitr)
  Integration Control/1 -> Integrator3/2

== system Global_Nocontrol/Wetland/Oxygen Control/0.25 ro 0.75 ==
  Inital Oxygen : Inport
  Integration Control : Inport  Port=2
  Constant : Inport  Port=3
  Ammonia k : Inport  Port=4
  K_nitr : Inport  Port=5
  " Nitrate" : MATLAB Function  TreatAsAtomicUnit=on
  " Oxygen Control" : MATLAB Function  TreatAsAtomicUnit=on
  Ammonia : Product
  Integrator3 : Integrator  ExternalReset=level hold  InitialConditionSource=external  InitialCondition=10
  Ammonia_k : Outport
  "Nitrate_k " : Outport  Port=2
  wires:
  Inital Oxygen/1 -> Integrator3/3
  " Nitrate"/1(K_Nitrate) -> "Nitrate_k "/1
  Ammonia/1 -> Ammonia_k/1
  Ammonia k/1 -> Ammonia/2
  Constant/1 -> " Oxygen Control"/2(K)
  " Oxygen Control"/1(dOxygen_Level) -> Integrator3/1
  Integrator3/1 -> " Oxygen Control"/1(c), " Nitrate"/1(Oxygen_Level), Ammonia/1
  K_nitr/1 -> " Nitrate"/2(K_Nitr)
  Integration Control/1 -> Integrator3/2

== system Global_Nocontrol/Wetland/Oxygen Control/0.75  ==
  Inital Oxygen : Inport
  Integration Control : Inport  Port=2
  Constant : Inport  Port=3
  Ammonia k : Inport  Port=4
  K_nitr : Inport  Port=5
  " Nitrate" : MATLAB Function  TreatAsAtomicUnit=on
  " Oxygen Control" : MATLAB Function  TreatAsAtomicUnit=on
  Ammonia : Product
  Integrator3 : Integrator  ExternalReset=level hold  InitialConditionSource=external  InitialCondition=10
  Ammonia_k : Outport
  "Nitrate_k " : Outport  Port=2
  wires:
  Inital Oxygen/1 -> Integrator3/3
  " Nitrate"/1(K_Nitrate) -> "Nitrate_k "/1
  Ammonia/1 -> Ammonia_k/1
  Ammonia k/1 -> Ammonia/2
  Constant/1 -> " Oxygen Control"/2(K)
  " Oxygen Control"/1(dOxygen_Level) -> Integrator3/1
  Integrator3/1 -> " Oxygen Control"/1(c), " Nitrate"/1(Oxygen_Level), Ammonia/1
  K_nitr/1 -> " Nitrate"/2(K_Nitr)
  Integration Control/1 -> Integrator3/2

== matlab function Global_Nocontrol/Wetland/ Ammonia - Nitrate - Interface ==
  data: C_am input; C_nit output; Cni input; Cam input
function C_nit = fcn(C_am,Cni,Cam)
C_nit=abs(C_am- Cam)+Cni;

== matlab function Global_Nocontrol/Wetland/ Ammonia and Nitrate  ==
  data: C1 input; C2 input; C3 input; v input; dc1 output; Cint input; Qi input; Qout input; dv input; k_am input; dc2 output; k_ni input; k_TSS input; dc3 output
function [dc1,dc2,dc3] = Nitrogen_Cycle(C1,C2,C3,v,Cint,Qi,Qout,dv,k_am,k_ni,k_TSS)

A=[Qi   0  0;
    0   Qi 0;
    0   0  Qi];

B=[Qout + dv + k_am    0               0;
    0              Qout + dv + k_ni    0;
    0                  0               Qout + dv + k_TSS ];

C=[C1;
   C2;
   C3];

if v==0
    dc1=0;
    dc2=0;
    dc3=0;
else 
    dc=(A*Cint - B*C)*(1/v);
    dc1=dc(1);
    dc2=dc(2);
    dc3=dc(3);

end

== matlab function Global_Nocontrol/Wetland/ Concentration  ==
  data: Nitrate input; Ammonia input; TSS input; C output; Qin input
function C = fcn(Nitrate,Ammonia,TSS,Qin)

if Qin>0
    C=[Ammonia; Nitrate;TSS];
else
    C=[0; 0; 0];
    
end

== matlab function Global_Nocontrol/Wetland/Height and Volume ==
  data: Qin input; A input; dH output; Qout input
function dH  = Height_and_Volume(Qin,A,Qout)
    dH = (Qin-Qout)*(1/A);
end

== matlab function Global_Nocontrol/Wetland/Overflow  ==
  data: H input; Q_overflow output; Qin input; Overflow_Height input
function Q_overflow = fcn(H,Qin,Overflow_Height)
%#codegen
if H>=Overflow_Height;
    Q_overflow= 2* (H-Overflow_Height);
else 
    Q_overflow=0;
end

== matlab function Global_Nocontrol/Wetland/Oxygen Control/ Oxygen Setpoint1 ==
  data: Height input; Intergration_Control output; Integration_Control1 output; Integration_Control2 output; Integration_Control3 output
function [Intergration_Control,Integration_Control1,Integration_Control2,Integration_Control3] = fcn(Height)
if Height>0 
    Intergration_Control=0;
else 
    Intergration_Control=1;
end
    
if Height>0.25
    Integration_Control1=0;
else 
    Integration_Control1=1;
end
if Height>0.75
    Integration_Control2=0;
else 
    Integration_Control2=1;
end
   
if Height>1.5
    Integration_Control3=0;
else 
    Integration_Control3=1;
end

== matlab function Global_Nocontrol/Wetland/Oxygen Control/0 to 0.25/ Nitrate ==
  data: Oxygen_Level input; K_Nitrate output; K_Nitr input
function K_Nitrate = fcn(Oxygen_Level,K_Nitr)

if Oxygen_Level< 1.0
    K_Nitrate = K_Nitr;
else
    K_Nitrate = 0;
end

== matlab function Global_Nocontrol/Subsystem1/ Ammonia - Nitrate - Interface ==
  data: C_am input; C_nit output; Cni input; Cam input
function C_nit = fcn(C_am,Cni,Cam)
C_nit=abs(C_am- Cam)+Cni;

== matlab function Global_Nocontrol/Subsystem1/ Ammonia and Nitrate  ==
  data: C1 input; C2 input; C3 input; v input; dc1 output; Cint input; Qi input; Qout input; dv input; k_am input; dc2 output; k_ni input; k_TSS input; dc3 output
function [dc1,dc2,dc3] = Nitrogen_Cycle(C1,C2,C3,v,Cint,Qi,Qout,dv,k_am,k_ni,k_TSS)

A=[Qi   0  0;
    0   Qi 0;
    0   0  Qi];

B=[Qout + dv + k_am    0               0;
    0              Qout + dv + k_ni    0;
    0                  0               Qout + dv + k_TSS ];

C=[C1;
   C2;
   C3];

if v==0
    dc1=0;
    dc2=0;
    dc3=0;
else 
    dc=(A*Cint - B*C)*(1/v);
    dc1=dc(1);
    dc2=dc(2);
    dc3=dc(3);

end

== matlab function Global_Nocontrol/Subsystem1/ Concentration  ==
  data: Nitrate input; Ammonia input; TSS input; C output; Qin input
function C = fcn(Nitrate,Ammonia,TSS,Qin)

if Qin>0
    C=[Ammonia; Nitrate;TSS];
else
    C=[0; 0; 0];
    
end

== matlab function Global_Nocontrol/Subsystem1/Height and Volume ==
  data: Qin input; A input; dH output; Qout input
function dH  = Height_and_Volume(Qin,A,Qout)
    dH = (Qin-Qout)*(1/A);
end

== matlab function Global_Nocontrol/Subsystem1/Overflow  ==
  data: H input; Q_overflow output; Qin input; Overflow_Height input
function Q_overflow = fcn(H,Qin,Overflow_Height)
%#codegen
if H>=Overflow_Height;
    Q_overflow=Qin;
else 
    Q_overflow=0;
end

== matlab function Global_Nocontrol/Subsystem1/Oxygen Control/ Oxygen Setpoint1 ==
  data: Height input; Intergration_Control output; Integration_Control1 output; Integration_Control2 output
function [Intergration_Control,Integration_Control1,Integration_Control2] = fcn(Height)
if Height>0 
    Intergration_Control=0;
else 
    Intergration_Control=1;
end
    
if Height>0.25
    Integration_Control1=0;
else 
    Integration_Control1=1;
end
if Height>0.75
    Integration_Control2=0;
else 
    Integration_Control2=1;
end

== matlab function Global_Nocontrol/Wetland/Oxygen Control/0 to 0.25/ Oxygen Control ==
  data: c input; dOxygen_Level output; K input
function dOxygen_Level = fcn(c,K)

dOxygen_Level = -c * K;

== matlab function Global_Nocontrol/Subsystem1/Oxygen Control/0 to 0.25/ Nitrate ==
  data: Oxygen_Level input; K_Nitrate output; K_Nitr input
function K_Nitrate = fcn(Oxygen_Level,K_Nitr)

if Oxygen_Level< 1.0
    K_Nitrate = K_Nitr;
else
    K_Nitrate = 0;
end

== matlab function Global_Nocontrol/Wetland/Q out ==
  data: H input; Qout output; Control_Height input; Weir_height input
function Qout = fcn(H,Control_Height,Weir_height)

if H<=Control_Height || H<Weir_height;
    Qout=0;
else
    Qout=sqrt(2*9.81*(H-Weir_height));
end

== matlab function Global_Nocontrol/Subsystem1/Oxygen Control/0 to 0.25/ Oxygen Control ==
  data: c input; dOxygen_Level output; K input
function dOxygen_Level = fcn(c,K)

dOxygen_Level = -c * K;

== matlab function Global_Nocontrol/Subsystem1/Q out ==
  data: H input; Qout output; Control_Height input
function Qout = fcn(H,Control_Height)

if H<=Control_Height
    Qout=0;
else
    
   Qout = sqrt(2*9.81*H);
   

end

== matlab function Global_Nocontrol/Subsystem3/ Ammonia - Nitrate - Interface ==
  data: C_am input; C_nit output; Cni input; Cam input
function C_nit = fcn(C_am,Cni,Cam)
C_nit=abs(C_am- Cam)+Cni;

== matlab function Global_Nocontrol/Subsystem3/ Ammonia and Nitrate  ==
  data: C1 input; C2 input; C3 input; v input; dc1 output; Cint input; Qi input; Qout input; dv input; k_am input; dc2 output; k_ni input; k_TSS input; dc3 output
function [dc1,dc2,dc3] = Nitrogen_Cycle(C1,C2,C3,v,Cint,Qi,Qout,dv,k_am,k_ni,k_TSS)

A=[Qi   0  0;
    0   Qi 0;
    0   0  Qi];

B=[Qout + dv + k_am    0               0;
    0              Qout + dv + k_ni    0;
    0                  0               Qout + dv + k_TSS ];

C=[C1;
   C2;
   C3];

if v==0
    dc1=0;
    dc2=0;
    dc3=0;
else 
    dc=(A*Cint - B*C)*(1/v);
    dc1=dc(1);
    dc2=dc(2);
    dc3=dc(3);

end

== matlab function Global_Nocontrol/Subsystem3/ Concentration  ==
  data: Nitrate input; Ammonia input; TSS input; C output; Qin input
function C = fcn(Nitrate,Ammonia,TSS,Qin)

if Qin>0
    C=[Ammonia; Nitrate;TSS];
else
    C=[0; 0; 0];
    
end

== matlab function Global_Nocontrol/Subsystem3/Height and Volume ==
  data: Qin input; A input; dH output; Qout input
function dH  = Height_and_Volume(Qin,A,Qout)
    dH = (Qin-Qout)*(1/A);
end

== matlab function Global_Nocontrol/Subsystem3/Overflow  ==
  data: H input; Q_overflow output; Qin input; Overflow_Height input
function Q_overflow = fcn(H,Qin,Overflow_Height)
%#codegen
if H>=Overflow_Height;
    Q_overflow=Qin;
else 
    Q_overflow=0;
end

== matlab function Global_Nocontrol/Subsystem3/Oxygen Control/ Oxygen Setpoint1 ==
  data: Height input; Intergration_Control output; Integration_Control1 output; Integration_Control2 output
function [Intergration_Control,Integration_Control1,Integration_Control2] = fcn(Height)
if Height>0 
    Intergration_Control=0;
else 
    Intergration_Control=1;
end
    
if Height>0.25
    Integration_Control1=0;
else 
    Integration_Control1=1;
end
if Height>0.75
    Integration_Control2=0;
else 
    Integration_Control2=1;
end

== matlab function Global_Nocontrol/Subsystem3/Oxygen Control/0 to 0.25/ Nitrate ==
  data: Oxygen_Level input; K_Nitrate output; K_Nitr input
function K_Nitrate = fcn(Oxygen_Level,K_Nitr)

if Oxygen_Level< 1.0
    K_Nitrate = K_Nitr;
else
    K_Nitrate = 0;
end

== matlab function Global_Nocontrol/Subsystem3/Oxygen Control/0 to 0.25/ Oxygen Control ==
  data: c input; dOxygen_Level output; K input
function dOxygen_Level = fcn(c,K)

dOxygen_Level = -c * K;

== matlab function Global_Nocontrol/Subsystem3/Q out ==
  data: H input; Qout output; Control_Height input
function Qout = fcn(H,Control_Height)

if H<=Control_Height
    Qout=0;
else
    
   Qout = sqrt(2*9.81*H);
   

end

== matlab function Global_Nocontrol/MATLAB Function ==
  data: q1 input; q output; q2 input; q3 input; c1 input; c2 input; c output; c3 input
function [q,c] = fcn(q1,q2,q3,c1,c2,c3)
%#codegen
if q1+q2+q3==0
    c=0;
    q=0;
else
    c=(c1*q1+c2*q2+q3*c3)/(q1+q2+q3); % Concentration computed using loads
    q=q1+q2+q3; % Sum of flows
end
end

== matlab function Global_Nocontrol/Subsystem2/ Ammonia - Nitrate - Interface ==
  data: C_am input; C_nit output; Cni input; Cam input
function C_nit = fcn(C_am,Cni,Cam)
C_nit=abs(C_am- Cam)+Cni;

== matlab function Global_Nocontrol/Subsystem2/ Ammonia and Nitrate  ==
  data: C1 input; C2 input; C3 input; v input; dc1 output; Cint input; Qi input; Qout input; dv input; k_am input; dc2 output; k_ni input; k_TSS input; dc3 output
function [dc1,dc2,dc3] = Nitrogen_Cycle(C1,C2,C3,v,Cint,Qi,Qout,dv,k_am,k_ni,k_TSS)

A=[Qi   0  0;
    0   Qi 0;
    0   0  Qi];

B=[Qout + dv + k_am    0               0;
    0              Qout + dv + k_ni    0;
    0                  0               Qout + dv + k_TSS ];

C=[C1;
   C2;
   C3];

if v==0
    dc1=0;
    dc2=0;
    dc3=0;
else 
    dc=(A*Cint - B*C)*(1/v);
    dc1=dc(1);
    dc2=dc(2);
    dc3=dc(3);

end

== matlab function Global_Nocontrol/Subsystem2/ Concentration  ==
  data: Nitrate input; Ammonia input; TSS input; C output; Qin input
function C = fcn(Nitrate,Ammonia,TSS,Qin)

if Qin>0
    C=[Ammonia; Nitrate;TSS];
else
    C=[0; 0; 0];
    
end
